simulink model "simul"  (Simulink 6.4)
settings: Solver=ode4  StartTime=0.0  StopTime=cas_simulacie  FixedStep=ptv_sim_step  RelTol=1e-3
values from neighbouring files (symbols this model uses):
  M = (y_max-y_min)/y_max    [km_id.m]    (also in km_sustavy.m)
  t_d = (ref(2)-a(1)-a(2)*s0)/z_r    [mup.m]    (also in nm.m = (a(3)^2)/(alfa*a(3)-a(2))/(Kv*z_r))
  t_i = 1e10    (= 10000000000)    [mup.m]    (also in nm.m)
  z_r = (ref(1)-a(1)*s0)/Kv    [mup.m]    (also in nm.m = ( ( ( ( a(2) + ( ( a(3)^2 ) / (alfa*a(4)) -a(2) ) )^2 ) / ( )
undefined symbols (not defined in the file or in its folder): b_w, C, Dr, presnost_riadenia, q_de, q_du, q_u, R_cas_zmeny, R_nova, R_povodna, t_f, t_r, U_dolne_obmedzenie, U_horne_obmedzenie, W_cas_zmeny, W_nova, W_povodna
settings Model: Creator=oravec  LastModifiedBy=oravec
settings OptimizationCC: InitFltsAndDblsToZero=off
settings DebuggingCC: SignalResolutionControl=UseLocalSettings  MultiTaskDSMMsg=error  MultiTaskCondExecSysMsg=error  StrictBusMsg=ErrorLevel1
settings HardwareCC: TargetHWDeviceType=32-bit Generic

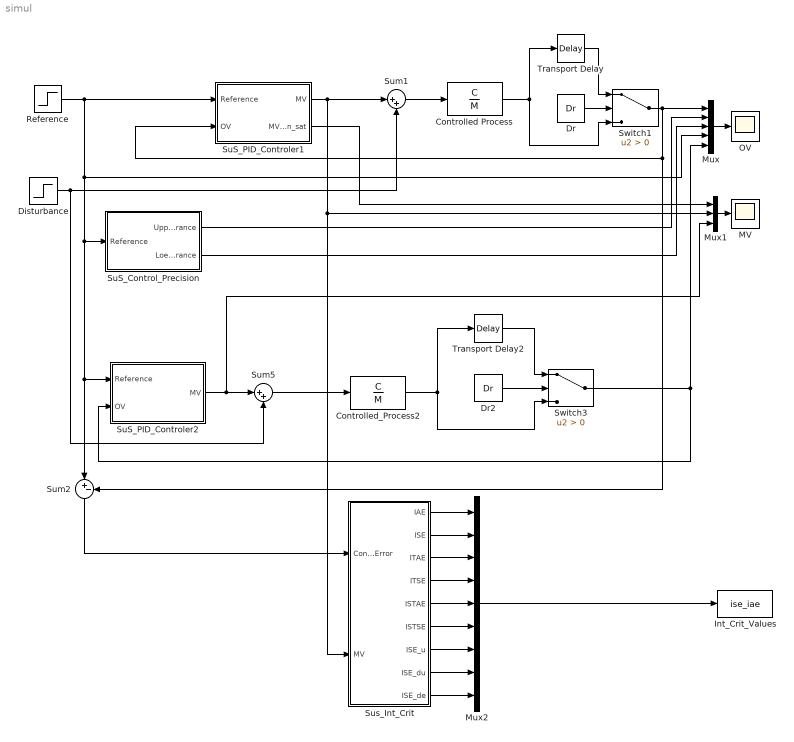
== system simul ==
  Controlled Process : TransferFcn  Numerator=C  Denominator=M
  Controlled_Process2 : TransferFcn  Numerator=C  Denominator=M
  Disturbance : Step  Time=R_cas_zmeny  Before=R_povodna  After=R_nova  SampleTime=0
  Dr : Constant  Value=Dr
  Dr2 : Constant  Value=Dr
  Int_Crit_Values : ToWorkspace  VariableName=ise_iae  SampleTime=-1  SaveFormat=Array
      settings: MaxDataPoints=1
  MV : Scope
      settings: SaveName=akcnavel  DataFormat=Array
  Mux : Mux  Inputs=5
  Mux1 : Mux  Inputs=3
  Mux2 : Mux  Inputs=9
  OV : Scope
      settings: TimeRange=50  SaveName=sim_data  DataFormat=Array
  Reference : Step  Time=W_cas_zmeny  Before=W_povodna  After=W_nova  SampleTime=0
  SuS_Control_Precision : Subsystem
  SuS_PID_Controler1 : Subsystem
  SuS_PID_Controler2 : Subsystem
  Sum1 : Sum  Inputs=|++  SaturateOnIntegerOverflow=on
  Sum2 : Sum  Orientation=down  Inputs=|+-  SaturateOnIntegerOverflow=on
  Sum5 : Sum  Inputs=|++  SaturateOnIntegerOverflow=on
  Sus_Int_Crit : Subsystem
  Switch1 : Switch  Criteria=u2 > Threshold
  Switch3 : Switch  Criteria=u2 > Threshold
  Transport Delay : TransportDelay  DelayTime=Dr
  Transport Delay2 : TransportDelay  DelayTime=Dr
  wires:
  Reference/1 -> Mux/4, SuS_Control_Precision/1(Reference), Sum2/1, SuS_PID_Controler2/1(Reference), SuS_PID_Controler1/1(Reference)
  SuS_PID_Controler1/1(MV) -> Sum1/1, Mux1/2, Sus_Int_Crit/2(MV)
  Dr/1 -> Switch1/2
  Controlled Process/1 -> Transport Delay/1, Switch1/3
  Transport Delay/1 -> Switch1/1
  Switch1/1 -> Mux/1, SuS_PID_Controler1/2(OV), Sum2/2
  Mux/1 -> OV/1
  SuS_Control_Precision/1(Upper_Tolerance) -> Mux/2
  SuS_Control_Precision/2(Loewr_Tolerance) -> Mux/3
  Disturbance/1 -> Sum1/2, Sum5/2
  Dr2/1 -> Switch3/2
  Controlled_Process2/1 -> Transport Delay2/1, Switch3/3
  Transport Delay2/1 -> Switch3/1
  Switch3/1 -> Mux/5, SuS_PID_Controler2/2(OV)
  Mux1/1 -> MV/1
  SuS_PID_Controler1/2(MV_non_sat) -> Mux1/1
  SuS_PID_Controler2/1(MV) -> Sum5/1, Mux1/3
  Sum5/1 -> Controlled_Process2/1
  Sum1/1 -> Controlled Process/1
  Sum2/1 -> Sus_Int_Crit/1(Control_Error)
  Sus_Int_Crit/1(IAE) -> Mux2/1
  Sus_Int_Crit/2(ISE) -> Mux2/2
  Sus_Int_Crit/3(ITAE) -> Mux2/3
  Sus_Int_Crit/4(ITSE) -> Mux2/4
  Sus_Int_Crit/5(ISTAE) -> Mux2/5
  Sus_Int_Crit/6(ISTSE) -> Mux2/6
  Sus_Int_Crit/7(ISE_u) -> Mux2/7
  Sus_Int_Crit/8(ISE_du) -> Mux2/8
  Sus_Int_Crit/9(ISE_de) -> Mux2/9
  Mux2/1 -> Int_Crit_Values/1

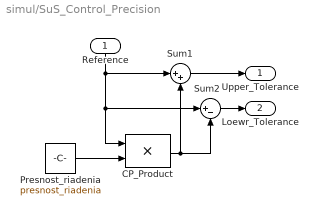
== system simul/SuS_Control_Precision ==
  Reference : Inport  Orientation=down
  CP_Product : Product  SaturateOnIntegerOverflow=on
  Presnost_riadenia : Constant  Value=presnost_riadenia
  Sum1 : Sum  Inputs=|++  SaturateOnIntegerOverflow=on
  Sum2 : Sum  Inputs=|+-  SaturateOnIntegerOverflow=on
  Upper_Tolerance : Outport
  Loewr_Tolerance : Outport  Port=2
  wires:
  Presnost_riadenia/1 -> CP_Product/2
  CP_Product/1 -> Sum1/2, Sum2/2
  Reference/1 -> Sum1/1, CP_Product/1, Sum2/1
  Sum1/1 -> Upper_Tolerance/1
  Sum2/1 -> Loewr_Tolerance/1

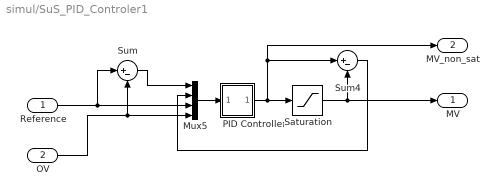
== system simul/SuS_PID_Controler1 ==
  Reference : Inport
  OV : Inport  Port=2
  Mux5 : Mux
  PID Controller : Subsystem  AncestorBlock=simulink_extras/Additional Linear/PID Controller  mask(PID Controller){P=z_r, I=z_r/t_i, D=z_r*t_d}
      mask prompts: P "Proportional:"; I "Integral:"; D "Derivative:"
      mask help:
      | Enter expressions for proportional, integral, and derivative terms.
      | P+I/s+Ds
      mask Help: This block implements a PID controller where parameters are entered for the Proportional, Integral and Derivative terms. Unmask this block to see how it works. The derivative term is implemented using a true derivative block.
      mask Display: disp('PID')
  Saturation : Saturate  UpperLimit=U_horne_obmedzenie  LowerLimit=U_dolne_obmedzenie
  Sum : Sum  Inputs=|+-  SaturateOnIntegerOverflow=on
  Sum4 : Sum  Inputs=|+-  SaturateOnIntegerOverflow=on
  MV : Outport
  MV_non_sat : Outport  Port=2
  wires:
  Mux5/1 -> PID Controller/1(In_1)
  PID Controller/1(Out_1) -> Saturation/1, Sum4/1, MV_non_sat/1
  Saturation/1 -> Sum4/2, MV/1
  Sum4/1 -> Mux5/2
  Reference/1 -> Mux5/3, Sum/1
  OV/1 -> Mux5/4, Sum/2
  Sum/1 -> Mux5/1

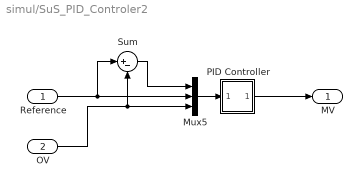
== system simul/SuS_PID_Controler2 ==
  Reference : Inport
  OV : Inport  Port=2
  Mux5 : Mux  Inputs=3
  PID Controller : Subsystem  AncestorBlock=simulink_extras/Additional Linear/PID Controller  mask(PID Controller){P=z_r, I=z_r/t_i, D=z_r*t_d}
      mask prompts: P "Proportional:"; I "Integral:"; D "Derivative:"
      mask help:
      | Enter expressions for proportional, integral, and derivative terms.
      | P+I/s+Ds
      mask Help: This block implements a PID controller where parameters are entered for the Proportional, Integral and Derivative terms. Unmask this block to see how it works. The derivative term is implemented using a true derivative block.
      mask Display: disp('PID')
  Sum : Sum  Inputs=|+-  SaturateOnIntegerOverflow=on
  MV : Outport
  wires:
  Sum/1 -> Mux5/1
  OV/1 -> Sum/2, Mux5/3
  Reference/1 -> Sum/1, Mux5/2
  PID Controller/1(Out_1) -> MV/1
  Mux5/1 -> PID Controller/1(In_1)

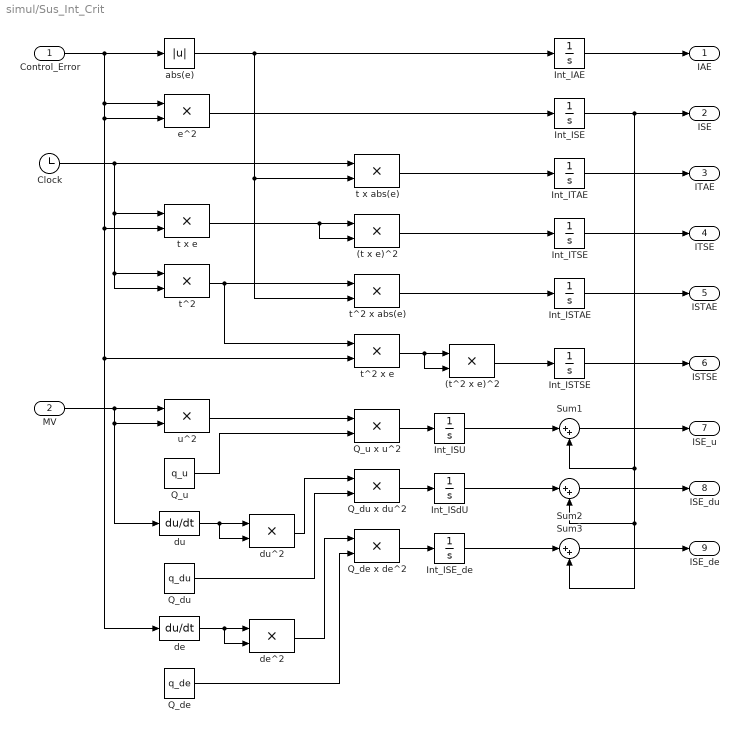
== system simul/Sus_Int_Crit ==
  Control_Error : Inport
  MV : Inport  Port=2
  (t x e)^2 : Product  SaturateOnIntegerOverflow=on
  (t^2 x e)^2 : Product  SaturateOnIntegerOverflow=on
  Clock : Clock
      settings: Decimation=10
  Int_IAE : Integrator
  Int_ISE : Integrator
  Int_ISE_de : Integrator
  Int_ISTAE : Integrator
  Int_ISTSE : Integrator
  Int_ISU : Integrator
  Int_ISdU : Integrator
  Int_ITAE : Integrator
  Int_ITSE : Integrator
  Q_de : Constant  Value=q_de
  Q_de x de^2 : Product  SaturateOnIntegerOverflow=on
  Q_du : Constant  Value=q_du
  Q_du x du^2 : Product  SaturateOnIntegerOverflow=on
  Q_u : Constant  Value=q_u
  Q_u x u^2 : Product  SaturateOnIntegerOverflow=on
  Sum1 : Sum  Inputs=|++  SaturateOnIntegerOverflow=on
  Sum2 : Sum  Inputs=|++  SaturateOnIntegerOverflow=on
  Sum3 : Sum  Inputs=|++  SaturateOnIntegerOverflow=on
  abs(e) : Abs  SaturateOnIntegerOverflow=on
  de : Derivative
  de^2 : Product  SaturateOnIntegerOverflow=on
  du : Derivative
  du^2 : Product  SaturateOnIntegerOverflow=on
  e^2 : Product  SaturateOnIntegerOverflow=on
  t x abs(e) : Product  SaturateOnIntegerOverflow=on
  t x e : Product  SaturateOnIntegerOverflow=on
  t^2 : Product  SaturateOnIntegerOverflow=on
  t^2 x abs(e) : Product  SaturateOnIntegerOverflow=on
  t^2 x e : Product  SaturateOnIntegerOverflow=on
  u^2 : Product  SaturateOnIntegerOverflow=on
  IAE : Outport
  ISE : Outport  Port=2
  ITAE : Outport  Port=3
  ITSE : Outport  Port=4
  ISTAE : Outport  Port=5
  ISTSE : Outport  Port=6
  ISE_u : Outport  Port=7
  ISE_du : Outport  Port=8
  ISE_de : Outport  Port=9
  wires:
  Int_ISTSE/1 -> ISTSE/1
  Int_ISTAE/1 -> ISTAE/1
  Int_ITSE/1 -> ITSE/1
  Int_ITAE/1 -> ITAE/1
  Int_IAE/1 -> IAE/1
  Q_de x de^2/1 -> Int_ISE_de/1
  Q_de/1 -> Q_de x de^2/2
  de^2/1 -> Q_de x de^2/1
  de/1 -> de^2/2, de^2/1
  Q_du/1 -> Q_du x du^2/2
  du^2/1 -> Q_du x du^2/1
  du/1 -> du^2/2, du^2/1
  Sum2/1 -> ISE_du/1
  Q_u/1 -> Q_u x u^2/2
  u^2/1 -> Q_u x u^2/1
  MV/1 -> du/1, u^2/2, u^2/1
  Sum1/1 -> ISE_u/1
  t^2 x abs(e)/1 -> Int_ISTAE/1
  t^2/1 -> t^2 x e/1, t^2 x abs(e)/1
  (t x e)^2/1 -> Int_ITSE/1
  Clock/1 -> t x abs(e)/1, t^2/2, t^2/1, t x e/1
  t x abs(e)/1 -> Int_ITAE/1
  Int_ISE/1 -> ISE/1, Sum1/2, Sum2/2, Sum3/2
  e^2/1 -> Int_ISE/1
  abs(e)/1 -> t^2 x abs(e)/2, t x abs(e)/2, Int_IAE/1
  Control_Error/1 -> e^2/2, t x e/2, de/1, t^2 x e/2, e^2/1, abs(e)/1
  Q_u x u^2/1 -> Int_ISU/1
  Int_ISU/1 -> Sum1/1
  Q_du x du^2/1 -> Int_ISdU/1
  Int_ISdU/1 -> Sum2/1
  Int_ISE_de/1 -> Sum3/1
  Sum3/1 -> ISE_de/1
  t x e/1 -> (t x e)^2/1, (t x e)^2/2
  t^2 x e/1 -> (t^2 x e)^2/1, (t^2 x e)^2/2
  (t^2 x e)^2/1 -> Int_ISTSE/1

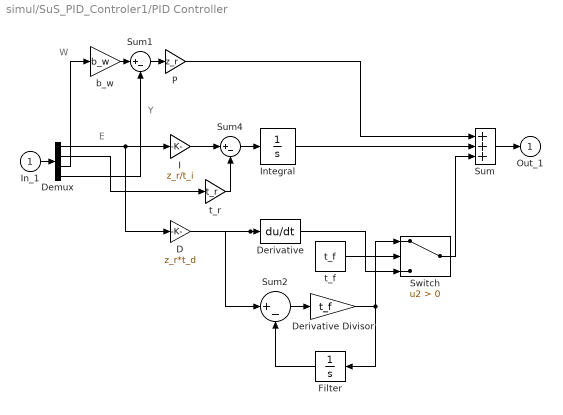
== system simul/SuS_PID_Controler1/PID Controller ==
  note: W
  note: Y
  note: E
  In_1 : Inport
  D : Gain  Gain=z_r*t_d  SaturateOnIntegerOverflow=on
  Demux : Demux
  Derivative : Derivative
  Derivative Divisor : Gain  Gain=t_f  SaturateOnIntegerOverflow=on
  Filter : Integrator  Orientation=left
  I : Gain  Gain=z_r/t_i  SaturateOnIntegerOverflow=on
  Integral : TransferFcn  Numerator=1  Denominator=[1 0]
  P : Gain  Gain=z_r  SaturateOnIntegerOverflow=on
  Sum : Sum  Inputs=+++  SaturateOnIntegerOverflow=on  InputSameDT=on
  Sum1 : Sum  Inputs=|+-  SaturateOnIntegerOverflow=on
  Sum2 : Sum  Inputs=|+-  SaturateOnIntegerOverflow=on  InputSameDT=on
  Sum4 : Sum  Inputs=|+-  SaturateOnIntegerOverflow=on
  Switch : Switch  Criteria=u2 > Threshold
  b_w : Gain  Gain=b_w  SaturateOnIntegerOverflow=on
  t_f : Constant  Value=t_f
  t_r : Gain  Gain=t_r  SaturateOnIntegerOverflow=on
  Out_1 : Outport  InitialOutput=0
  wires:
  D/1 -> Sum2/1, Derivative/1
  Sum/1 -> Out_1/1
  Integral/1 -> Sum/2
  P/1 -> Sum/1
  In_1/1 -> Demux/1
  Demux/1 -> D/1, I/1
  Sum4/1 -> Integral/1
  I/1 -> Sum4/1
  t_r/1 -> Sum4/2
  Demux/2 -> t_r/1
  Demux/3 -> b_w/1
  b_w/1 -> Sum1/1
  Sum1/1 -> P/1
  Demux/4 -> Sum1/2
  Filter/1 -> Sum2/2
  Derivative Divisor/1 -> Filter/1, Switch/1
  Sum2/1 -> Derivative Divisor/1
  t_f/1 -> Switch/2
  Switch/1 -> Sum/3
  Derivative/1 -> Switch/3

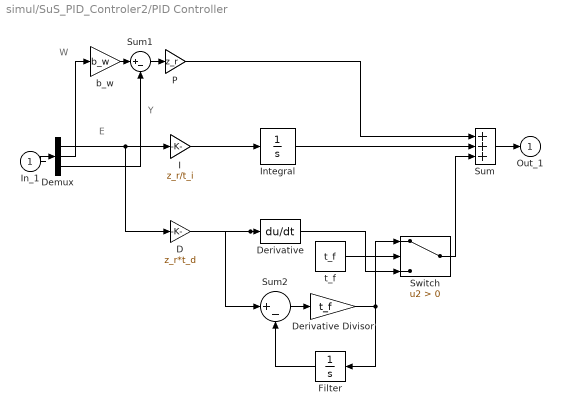
== system simul/SuS_PID_Controler2/PID Controller ==
  note: E
  note: Y
  note: W
  In_1 : Inport
  D : Gain  Gain=z_r*t_d  SaturateOnIntegerOverflow=on
  Demux : Demux  Outputs=3
  Derivative : Derivative
  Derivative Divisor : Gain  Gain=t_f  SaturateOnIntegerOverflow=on
  Filter : Integrator  Orientation=left
  I : Gain  Gain=z_r/t_i  SaturateOnIntegerOverflow=on
  Integral : TransferFcn  Numerator=1  Denominator=[1 0]
  P : Gain  Gain=z_r  SaturateOnIntegerOverflow=on
  Sum : Sum  Inputs=+++  SaturateOnIntegerOverflow=on  InputSameDT=on
  Sum1 : Sum  Inputs=|+-  SaturateOnIntegerOverflow=on
  Sum2 : Sum  Inputs=|+-  SaturateOnIntegerOverflow=on  InputSameDT=on
  Switch : Switch  Criteria=u2 > Threshold
  b_w : Gain  Gain=b_w  SaturateOnIntegerOverflow=on
  t_f : Constant  Value=t_f
  Out_1 : Outport  InitialOutput=0
  wires:
  Derivative/1 -> Switch/3
  Switch/1 -> Sum/3
  t_f/1 -> Switch/2
  Sum2/1 -> Derivative Divisor/1
  Derivative Divisor/1 -> Switch/1, Filter/1
  Filter/1 -> Sum2/2
  Sum1/1 -> P/1
  b_w/1 -> Sum1/1
  I/1 -> Integral/1
  Demux/1 -> I/1, D/1
  In_1/1 -> Demux/1
  P/1 -> Sum/1
  Integral/1 -> Sum/2
  Sum/1 -> Out_1/1
  D/1 -> Derivative/1, Sum2/1
  Demux/2 -> b_w/1
  Demux/3 -> Sum1/2
